simulink model "BDA_DynamicModel_pdg"  (R2021b)
settings: Solver=ode23t  StartTime=0.0  StopTime=10  FixedStep=0.000001  MaxStep=1e-5  MinStep=1e-7  RelTol=1e-3
undefined symbols (not defined in the file): X, Y, Z
libraries: sm_lib x47, nesl_utility x7, simulink x1
(part 2 of 3)

== matlab function BDA_DynamicModel_pdg/Modelo dinámico/h ==
  data: dq1 input; h output; dq2 input; dq3 input; dq4 input; dq5 input; dq6 input; q1 input; q2 input; q3 input; q4 input; q5 input; q6 input
function h = h(dq1,dq2,dq3,dq4,dq5,dq6,q1,q2,q3,q4,q5,q6)
%#codegen

%    This function was generated by the Symbolic Math Toolbox version 9.0.
%    01-Nov-2021 22:23:11

t2 = conj(dq1);
t3 = conj(dq2);
t4 = conj(dq3);
t5 = conj(dq4);
t6 = conj(dq5);
t7 = conj(dq6);
t8 = conj(q1);
t9 = conj(q2);
t10 = conj(q3);
t11 = conj(q4);
t12 = conj(q5);
t13 = conj(q6);
t14 = cos(q2);
t15 = cos(q4);
t16 = cos(q5);
t17 = cos(q6);
t18 = sin(q2);
t19 = sin(q4);
t20 = sin(q5);
t21 = sin(q6);
t22 = dq1+dq2;
t34 = dq5.*(3.0./5.0e+2);
t44 = dq3.*5.110348748545983e-1;
t51 = dq3.*8.595599785252598e-1;
t52 = dq5.*1.247162e-2;
t55 = 9.007199254740992e+15;
t56 = dq6.*9.99471e-3;
t58 = dq6.*1.838876e-2;
t60 = dq5.*5.68686e-3;
t63 = dq4.*5.84482e-3;
t67 = dq4.*6.47e-6;
t102 = dq3.*2.688673858077708e-3;
t103 = dq3.*2.986906857247653e-3;
t111 = dq3.*3.306395640309251e-6;
t23 = cos(t8);
t24 = cos(t9);
t25 = cos(t11);
t26 = cos(t12);
t27 = cos(t13);
t28 = sin(t8);
t29 = sin(t9);
t30 = sin(t11);
t31 = sin(t12);
t32 = sin(t13);
t33 = t2+t3;
t42 = t14.*1.051339e-1;
t43 = t18.*1.051339e-1;
t45 = t4.*5.110348748545983e-1;
t46 = t16.*5.110348748545983e-1;
t48 = t20.*5.110348748545983e-1;
t53 = t18.*3.235525e-2;
t54 = t4.*8.595599785252598e-1;
t59 = t14.*3.235525e-2;
t64 = t16.*t19.*8.595599785252598e-1;
t65 = t19.*t20.*8.595599785252598e-1;
t68 = t6.*4.36041e-5;
t69 = t6.*5.58e-9;
t70 = t6.*6.12e-9;
t71 = t6.*1.247162e-10;
t72 = t6.*5.68686e-11;
t73 = t6.*5.4e-10;
t75 = (q3.*t55)./9.007199254740992e+15;
t76 = (t10.*t55)./9.007199254740992e+15;
t81 = q3.*t55.*1.110223024625157e-16i;
t82 = t10.*t55.*1.110223024625157e-16i;
t104 = t7.*1.33637554986e-4;
t105 = t5.*1.688944904408e-4;
t106 = t7.*7.26350557185e-5;
t107 = t6.*6.1855407534e-5;
t109 = t6.*1.35652563578e-4;
t110 = t15.*t16.*4.990257941055339e-2;
t114 = t6.*7.732404399999999e-9;
t116 = t6.*3.5258532e-9;
t117 = t5.*1.869599668e-7;
t118 = t7.*1.87565352e-8;
t119 = t5.*4.57649406e-8;
t121 = t7.*1.01946042e-8;
t123 = t5.*6.36648e-11;
t124 = t5.*1.89372168e-8;
t125 = t5.*1.81773902e-8;
t127 = t6.*3.740375e-9;
t128 = t6.*3.2206632e-9;
t129 = t7.*1.96560591e-8;
t130 = t7.*1.09500687e-8;
t131 = t5.*2.01217e-11;
t132 = t5.*2.09628e-11;
t147 = t4.*8.974336263707516e-6;
t159 = t4.*8.631097478604537e-5;
t160 = t4.*3.253493310064303e-11;
t163 = t4.*2.338748069224912e-8;
t164 = t4.*9.289280326040201e-9;
t165 = t4.*2.957541243885479e-10;
t166 = t4.*9.554306323645785e-8;
t168 = t4.*1.344336929038854e-10;
t170 = t4.*4.301878172924333e-10;
t171 = t4.*9.677578217482396e-9;
t173 = t4.*1.028289044136177e-11;
t176 = t4.*1.071272187460197e-11;
t35 = t23.*t24.*(9.81e+2./1.0e+2);
t36 = t23.*t29.*(9.81e+2./1.0e+2);
t37 = t24.*t28.*(9.81e+2./1.0e+2);
t38 = t28.*t29.*(9.81e+2./1.0e+2);
t47 = -t43;
t49 = t24.*1.051339e-1;
t50 = t29.*1.051339e-1;
t61 = t24.*3.235525e-2;
t62 = t29.*3.235525e-2;
t66 = -t65;
t74 = -t71;
t77 = cos(t75);
t78 = sin(t75);
t79 = cos(t76);
t80 = sin(t76);
t83 = exp(t81);
t84 = -t81;
t85 = -t82;
t89 = exp(t82);
t112 = t42+t53;
t122 = t48+t64;
t39 = -t38;
t40 = t36+t37;
t57 = -t50;
t86 = 1.0./t83;
t87 = t15.*t77;
t88 = t19.*t77;
t90 = exp(t85);
t91 = t83-1.0;
t94 = t22.*t25.*t79;
t96 = t22.*t30.*t79;
t113 = t47+t59;
t115 = t49+t62;
t126 = t46+t66;
t133 = t77.*1.025512e-2;
t134 = t77.*1.273194e-2;
t135 = t77.*9.224950000000001e-3;
t143 = t22.*t79.*1.273194e-2;
t144 = t22.*t79.*1.025512e-2;
t145 = t22.*t79.*9.224950000000001e-3;
t180 = t83.*3.694216783411725e-1;
t181 = t83.*1.305783216588275e-1;
t183 = t89.*1.305783216588275e-1;
t184 = t89.*3.694216783411725e-1;
t188 = t33.*t77.*3.42298471896e-5;
t189 = t33.*t77.*3.07913148585e-5;
t190 = t33.*t77.*1.252822896e-7;
t191 = t33.*t77.*3.679077402936e-4;
t196 = t33.*t77.*2.2561264e-9;
t200 = t33.*t77.*1.5275005e-9;
t202 = t33.*t77.*2.029489e-9;
t203 = t33.*t77.*9.96910902e-8;
t204 = t33.*t77.*4.12514856e-8;
t208 = t33.*t77.*2.1020667e-9;
t226 = t15.*t55.*t78.*5.673626844500105e-17;
t227 = t19.*t55.*t78.*5.673626844500105e-17;
t228 = t16.*t55.*t78.*9.543032792050485e-17;
t229 = t20.*t55.*t78.*9.543032792050485e-17;
t232 = t22.*t55.*t80.*5.673626844500105e-17;
t233 = t22.*t55.*t80.*9.543032792050485e-17;
t234 = t15.*t55.*t78.*3.404176106700063e-19;
t236 = t33.*t55.*t78.*5.673626844500105e-17;
t237 = t33.*t55.*t78.*9.543032792050485e-17;
t239 = t83.*3.215186923359161e-3;
t241 = t83.*1.345257168956303e-2;
t242 = t89.*3.215186923359161e-3;
t243 = t89.*1.345257168956303e-2;
t247 = t55.*t78.*4.87211480085e-18;
t250 = t20.*t55.*t78.*9.537984527703491e-19;
t252 = t55.*t78.*5.577730892363251e-19;
t253 = t22.*t55.*t80.*4.87211480085e-18;
t254 = t20.*t55.*t78.*1.754845396851463e-18;
t255 = t15.*t55.*t78.*7.075931802640439e-19;
t256 = t15.*t55.*t78.*2.479366200131245e-18;
t258 = t15.*t55.*t78.*3.226512155691387e-19;
t259 = t20.*t55.*t78.*5.426989146380022e-19;
t260 = t19.*t55.*t78.*3.31613276532711e-19;
t261 = t16.*t55.*t78.*1.190170786299927e-18;
t262 = t15.*t55.*t78.*7.351481000981246e-18;
t263 = t19.*t55.*t78.*9.810473427588925e-18;
t264 = t19.*t55.*t78.*4.938358626738924e-18;
t265 = t22.*t55.*t80.*6.374153504905841e-18;
t270 = t16.*t55.*t78.*6.183885249248715e-21;
t272 = t20.*t55.*t78.*6.183885249248715e-21;
t273 = t55.*t78.*6.174342216456664e-22;
t274 = t22.*t55.*t80.*5.577730892363251e-19;
t275 = t15.*t55.*t78.*3.670836568391568e-22;
t278 = t22.*t55.*t80.*6.174342216456664e-22;
t304 = t33.*t55.*t78.*2.127584079327986e-20;
t309 = t33.*t55.*t78.*1.611765660673211e-20;
t310 = t55.*t78.*t112.*5.673626844500105e-17;
t312 = t33.*t55.*t78.*1.807184809125693e-24;
t313 = t33.*t55.*t78.*4.367363288720426e-24;
t314 = t33.*t55.*t78.*7.011568855396425e-25;
t316 = t33.*t55.*t78.*3.18707675245292e-25;
t317 = t33.*t55.*t78.*6.075552740993358e-27;
t318 = t33.*t55.*t78.*1.78416509397307e-23;
t319 = t33.*t55.*t78.*1.019864560784935e-24;
t322 = t33.*t55.*t78.*1.734674307524971e-24;
t326 = t33.*t55.*t78.*2.000486878131959e-27;
t331 = t33.*t55.*t78.*1.920220429318022e-27;
t393 = t2.*t55.*t78.*t112.*1.893760189037778e-19;
t400 = t2.*t55.*t78.*t112.*6.240989528950116e-24;
t402 = t2.*t55.*t78.*t112.*2.836813422250052e-24;
t408 = t2.*t55.*t78.*t112.*9.077802951200168e-24;
t41 = t35+t39;
t92 = t91.^2;
t93 = t90-1.0;
t95 = t33.*t87;
t97 = t33.*t88;
t98 = t88.*(3.0./5.0e+2);
t100 = -t96;
t108 = t96.*(3.0./5.0e+2);
t120 = t57+t61;
t136 = t88.*2.228474e-2;
t137 = t87.*4.539638e-2;
t138 = t88.*4.539638e-2;
t139 = t88.*1.247162e-2;
t140 = t88.*5.68686e-3;
t141 = t87.*5.84482e-3;
t142 = t87.*6.562549e-2;
t146 = t33.*t134;
t148 = t88.*6.47e-6;
t149 = t96.*2.228474e-2;
t151 = t94.*4.539638e-2;
t152 = t96.*4.539638e-2;
t154 = t96.*1.247162e-2;
t155 = t94.*5.84482e-3;
t156 = t94.*6.562549e-2;
t158 = t96.*5.68686e-3;
t161 = t96.*6.47e-6;
t182 = t86.*3.694216783411725e-1;
t185 = t86.*1.305783216588275e-1;
t186 = t90.*1.305783216588275e-1;
t187 = t90.*3.694216783411725e-1;
t230 = -t227;
t231 = -t228;
t235 = -t232;
t238 = -t236;
t240 = t86.*3.215186923359161e-3;
t244 = t86.*1.345257168956303e-2;
t245 = t90.*3.215186923359161e-3;
t246 = t90.*1.345257168956303e-2;
t248 = t40.*t55.*t80.*5.673626844500105e-17;
t257 = t33.*t247;
t266 = -t260;
t267 = -t261;
t268 = -t263;
t269 = -t264;
t271 = -t265;
t276 = -t275;
t277 = t44+t233;
t281 = t45+t237;
t297 = t40.*t55.*t80.*1.893760189037778e-19;
t299 = t88+t226;
t307 = -t304;
t311 = t55.*t78.*t113.*9.543032792050485e-17;
t320 = t2.*t310;
t321 = -t314;
t323 = -t316;
t324 = -t319;
t327 = dq1.*t55.*t80.*t115.*5.673626844500105e-17;
t328 = t2.*t55.*t78.*t113.*(-9.543032792050485e-17);
t397 = -t393;
t399 = t2.*t55.*t78.*t113.*3.185302114428987e-19;
t403 = -t400;
t404 = t2.*t55.*t78.*t113.*1.049733607125553e-23;
t407 = -t402;
t409 = t2.*t55.*t78.*t113.*4.771516396025242e-24;
t412 = t2.*t55.*t78.*t113.*1.526885246728078e-23;
t418 = -t408;
t99 = t93.^2;
t101 = -t97;
t150 = t97.*2.228474e-2;
t153 = -t148;
t157 = t95.*6.562549e-2;
t162 = t97.*4.36041e-5;
t167 = -t161;
t169 = t97.*5.58e-9;
t172 = t97.*6.12e-9;
t174 = t97.*1.247162e-10;
t175 = t97.*5.68686e-11;
t177 = t95.*6.562549e-10;
t178 = t97.*5.4e-10;
t192 = t95.*4.467003792e-7;
t193 = t95.*1.3117937708872e-3;
t194 = t97.*1.3117937708872e-3;
t195 = t97.*1.35652563578e-4;
t197 = t95.*5.75130288e-8;
t198 = t95.*1.688944904408e-4;
t199 = t97.*6.1855407534e-5;
t201 = t95.*7.13801892181e-4;
t205 = t97.*3.554536554e-7;
t206 = t97.*7.732404399999999e-9;
t207 = t97.*1.869599668e-7;
t209 = t97.*1.411827418e-7;
t210 = t97.*1.470842712e-7;
t211 = t97.*3.5258532e-9;
t213 = t97.*6.36648e-11;
t214 = t95.*3.74065293e-8;
t216 = t95.*1.928492118e-7;
t217 = t95.*1.601199586e-7;
t218 = t95.*2.6250196e-9;
t219 = t95.*1.57501176e-8;
t220 = t97.*3.740375e-9;
t221 = t97.*3.2206632e-9;
t222 = t97.*5.06601e-11;
t223 = t97.*2.09628e-11;
t249 = t41.*t55.*t80.*9.543032792050485e-17;
t251 = -t248;
t279 = dq4+t277;
t280 = t51+t235;
t282 = t5+t281;
t283 = t54+t238;
t298 = -t297;
t300 = t41.*t55.*t80.*3.185302114428987e-19;
t301 = t87+t230;
t302 = t17.*t299;
t303 = t21.*t299;
t315 = -t311;
t325 = t2.*t311;
t329 = -t327;
t330 = dq1.*t55.*t80.*t120.*9.543032792050485e-17;
t332 = t86.*t92.*7.997968101822611e-3;
t334 = t25.*t277.*1.273194e-2;
t335 = t30.*t277.*1.273194e-2;
t337 = t15.*t281.*1.273194e-2;
t338 = t19.*t281.*1.273194e-2;
t340 = t86.*t92.*5.407940120688672e-3;
t369 = t19.*t281.*1.273194e-10;
t388 = t16.*t299.*4.334075e-2;
t389 = t20.*t299.*4.334075e-2;
t406 = t19.*t281.*1.252822896e-7;
t414 = t15.*t281.*3.679077402936e-4;
t415 = t19.*t281.*3.679077402936e-4;
t417 = t19.*t281.*1.38484038186e-4;
t436 = t15.*t281.*9.96910902e-8;
t438 = t15.*t281.*3.95963334e-8;
t439 = t19.*t281.*3.95963334e-8;
t442 = t19.*t281.*7.257205800000001e-9;
t453 = t15.*t281.*4.12514856e-8;
t455 = t19.*t281.*4.12514856e-8;
t463 = t19.*t281.*5.092776e-10;
t465 = t19.*t281.*3.0556656e-9;
t484 = t86.*t92.*t112.*2.196325630278387e-1;
t495 = t86.*t92.*t113.*2.196325630278387e-1;
t509 = t2.*t86.*t92.*t113.*(-2.196325630278387e-1);
t521 = t2.*t86.*t92.*t112.*7.330961578512107e-4;
t528 = t2.*t86.*t92.*t113.*7.330961578512107e-4;
t529 = t2.*t86.*t92.*t112.*6.346599179580158e-3;
t537 = t2.*t86.*t92.*t112.*2.161184420193933e-6;
t538 = t2.*t86.*t92.*t112.*7.116095042101973e-7;
t539 = t2.*t86.*t92.*t112.*1.719722968507977e-6;
t540 = t2.*t86.*t92.*t112.*4.831916386612451e-8;
t541 = t2.*t86.*t92.*t112.*1.098162815139193e-8;
t542 = t2.*t86.*t92.*t113.*2.415958193306225e-8;
t543 = t2.*t86.*t92.*t113.*4.831916386612451e-8;
t544 = t2.*t86.*t92.*t112.*3.514121008445419e-8;
t547 = t2.*t86.*t92.*t113.*1.098162815139193e-8;
t555 = t180+t182+2.61156643317655e-1;
t556 = t181+t185+7.38843356682345e-1;
t557 = t183+t186+7.38843356682345e-1;
t558 = t184+t187+2.61156643317655e-1;
t714 = t257+t320+t328;
t777 = t147+t307+t397+t399;
t778 = t165+t321+t403+t404;
t779 = t168+t323+t407+t409;
t780 = t170+t324+t412+t418;
t179 = -t174;
t212 = -t207;
t215 = -t213;
t224 = -t222;
t225 = -t223;
t284 = t26.*t279;
t285 = t31.*t279;
t286 = t25.*t280;
t287 = t30.*t280;
t288 = t20.*t282;
t289 = t15.*t283;
t290 = t19.*t283;
t291 = t16.*t282;
t305 = t16.*t301;
t306 = t20.*t301;
t308 = -t303;
t333 = -t330;
t342 = -t335;
t343 = -t338;
t345 = t89.*t99.*7.997968101822611e-3;
t349 = t40.*t89.*t99.*2.196325630278387e-1;
t356 = t89.*t99.*5.407940120688672e-3;
t358 = t41.*t89.*t99.*2.196325630278387e-1;
t371 = -t369;
t386 = t303.*9.99471e-3;
t387 = t302.*1.838876e-2;
t401 = t40.*t89.*t99.*7.330961578512107e-4;
t405 = t41.*t89.*t99.*7.330961578512107e-4;
t411 = -t406;
t416 = t40.*t89.*t99.*6.346599179580158e-3;
t422 = -t415;
t423 = -t417;
t451 = -t439;
t456 = -t442;
t466 = -t455;
t477 = -t463;
t480 = -t465;
t501 = t2.*t484;
t503 = -t495;
t508 = t2.*t495;
t510 = dq1.*t89.*t99.*t115.*2.196325630278387e-1;
t511 = dq1.*t89.*t99.*t120.*2.196325630278387e-1;
t536 = -t528;
t548 = -t543;
t549 = -t542;
t553 = -t547;
t617 = t40.*t557;
t618 = t41.*t558;
t619 = t249+t251;
t620 = -t25.*(t248-t249);
t621 = -t30.*(t248-t249);
t633 = t112.*t556;
t634 = t113.*t555;
t635 = t25.*(t248-t249).*(-2.889644e-2);
t636 = t30.*(t248-t249).*(-2.889644e-2);
t640 = t30.*(t248-t249).*(-1.08769e-2);
t641 = dq1.*t115.*t557;
t643 = dq1.*t120.*t558;
t707 = t247+t310+t315;
t720 = t15.*t714;
t721 = t19.*t714;
t728 = t239+t240+t332+1.819229615328168e-2;
t729 = t241+t244+t340+9.510076620873934e-3;
t770 = t102+t271+t329+t330;
t796 = t277.*t778;
t797 = t277.*t779;
t798 = t280.*t779;
t799 = t280.*t780;
t292 = -t286;
t293 = -t289;
t294 = -t291;
t295 = t286.*(3.0./5.0e+2);
t336 = t285.*1.838876e-2;
t339 = t284.*1.247162e-2;
t341 = t285.*9.99471e-3;
t344 = t286.*2.228474e-2;
t347 = t286.*4.539638e-2;
t348 = t287.*4.539638e-2;
t350 = t285.*5.68686e-3;
t351 = t286.*1.247162e-2;
t352 = t284.*6.48e-5;
t353 = t286.*5.68686e-3;
t354 = t285.*6.48e-5;
t359 = -t349;
t360 = t289.*2.228474e-2;
t361 = t287.*5.84482e-3;
t362 = t287.*6.562549e-2;
t365 = t290.*6.562549e-2;
t366 = -t358;
t368 = t286.*6.47e-6;
t370 = t289.*4.36041e-5;
t373 = t289.*5.58e-9;
t375 = t289.*6.12e-9;
t376 = t289.*1.247162e-10;
t377 = t288.*5.68686e-11;
t378 = t289.*5.68686e-11;
t380 = t290.*6.562549e-10;
t381 = t289.*5.4e-10;
t385 = t288.*6.48e-13;
t390 = t305.*9.99471e-3;
t391 = t305.*1.838876e-2;
t392 = t306.*1.247162e-2;
t394 = t305.*5.68686e-3;
t395 = t305.*6.48e-5;
t396 = t306.*6.48e-5;
t410 = -t405;
t413 = t94+t287;
t419 = t290.*4.467003792e-7;
t420 = t289.*1.3117937708872e-3;
t421 = t290.*1.3117937708872e-3;
t424 = t95+t290;
t425 = t290.*5.75130288e-8;
t426 = t288.*7.26350557185e-5;
t427 = t290.*1.688944904408e-4;
t428 = t288.*6.1855407534e-5;
t430 = t289.*6.1855407534e-5;
t431 = t100+t286;
t432 = t291.*1.35652563578e-4;
t433 = t289.*1.35652563578e-4;
t434 = t288.*1.33637554986e-4;
t437 = t290.*7.13801892181e-4;
t443 = t101+t289;
t449 = t289.*3.554536554e-7;
t450 = t289.*7.732404399999999e-9;
t452 = t291.*7.0482312e-7;
t454 = t288.*7.0482312e-7;
t457 = t289.*1.470842712e-7;
t459 = t289.*3.5258532e-9;
t460 = t291.*7.1088234e-9;
t462 = t288.*3.2415102e-9;
t464 = t289.*1.869599668e-7;
t468 = t289.*1.411827418e-7;
t469 = t288.*4.0176e-11;
t470 = t288.*1.87565352e-8;
h = ft_1({dq1,dq5,dq6,t103,t104,t105,t106,t107,t108,t109,t110,t111,t112,t114,t116,t117,t118,t119,t121,t122,t123,t124,t125,t126,t127,t128,t129,t130,t131,t132,t133,t134,t135,t136,t137,t138,t139,t140,t141,t142,t143,t144,t145,t146,t149,t15,t150,t151,t152,t153,t154,t155,t156,t157,t158,t159,t16,t160,t162,t163,t164,t166,t167,t169,t17,t171,t172,t173,t174,t175,t176,t177,t178,t179,t188,t189,t19,t190,t191,t192,t193,t194,t195,t196,t197,t198,t199,t2,t20,t200,t201,t202,t203,t204,t205,t206,t208,t209,t21,t210,t211,t212,t214,t215,t216,t217,t218,t219,t22,t220,t221,t224,t225,t228,t229,t23,t231,t234,t24,t242,t243,t245,t246,t248,t249,t25,t250,t252,t253,t254,t255,t256,t258,t259,t26,t262,t266,t267,t268,t269,t27,t270,t272,t273,t274,t276,t277,t278,t279,t28,t280,t284,t285,t288,t289,t29,t290,t291,t292,t293,t294,t295,t297,t298,t299,t30,t300,t301,t302,t303,t305,t306,t308,t309,t31,t310,t312,t313,t315,t317,t318,t32,t322,t326,t327,t33,t331,t333,t334,t336,t337,t339,t34,t341,t342,t343,t344,t345,t347,t348,t349,t350,t351,t352,t353,t354,t356,t358,t359,t360,t361,t362,t365,t366,t368,t370,t371,t373,t375,t376,t377,t378,t380,t381,t385,t386,t387,t388,t389,t390,t391,t392,t394,t395,t396,t40,t401,t405,t41,t410,t411,t413,t414,t416,t419,t420,t421,t422,t423,t424,t425,t426,t427,t428,t43,t430,t432,t433,t434,t436,t437,t438,t449,t450,t451,t452,t453,t454,t456,t457,t459,t460,t462,t464,t466,t468,t469,t470,t477,t480,t484,t501,t503,t509,t510,t511,t52,t521,t529,t536,t537,t538,t539,t540,t541,t544,t548,t549,t55,t553,t56,t58,t59,t6,t60,t617,t618,t620,t621,t63,t633,t634,t635,t636,t640,t641,t643,t67,t68,t69,t70,t707,t71,t72,t720,t721,t728,t729,t73,t74,t77,t770,t777,t78,t79,t796,t797,t798,t799,t80,t96,t97,t98});
end
function h = ft_1(ct)
dq1 = ct{1};
dq5 = ct{2};
dq6 = ct{3};
t103 = ct{4};
t104 = ct{5};
t105 = ct{6};
t106 = ct{7};
t107 = ct{8};
t108 = ct{9};
t109 = ct{10};
t110 = ct{11};
t111 = ct{12};
t112 = ct{13};
t114 = ct{14};
t116 = ct{15};
t117 = ct{16};
t118 = ct{17};
t119 = ct{18};
t121 = ct{19};
t122 = ct{20};
t123 = ct{21};
t124 = ct{22};
t125 = ct{23};
t126 = ct{24};
t127 = ct{25};
t128 = ct{26};
t129 = ct{27};
t130 = ct{28};
t131 = ct{29};
t132 = ct{30};
t133 = ct{31};
t134 = ct{32};
t135 = ct{33};
t136 = ct{34};
t137 = ct{35};
t138 = ct{36};
t139 = ct{37};
t140 = ct{38};
t141 = ct{39};
t142 = ct{40};
t143 = ct{41};
t144 = ct{42};
t145 = ct{43};
t146 = ct{44};
t149 = ct{45};
t15 = ct{46};
t150 = ct{47};
t151 = ct{48};
t152 = ct{49};
t153 = ct{50};
t154 = ct{51};
t155 = ct{52};
t156 = ct{53};
t157 = ct{54};
t158 = ct{55};
t159 = ct{56};
t16 = ct{57};
t160 = ct{58};
t162 = ct{59};
t163 = ct{60};
t164 = ct{61};
t166 = ct{62};
t167 = ct{63};
t169 = ct{64};
t17 = ct{65};
t171 = ct{66};
t172 = ct{67};
t173 = ct{68};
t174 = ct{69};
t175 = ct{70};
t176 = ct{71};
t177 = ct{72};
t178 = ct{73};
t179 = ct{74};
t188 = ct{75};
t189 = ct{76};
t19 = ct{77};
t190 = ct{78};
t191 = ct{79};
t192 = ct{80};
t193 = ct{81};
t194 = ct{82};
t195 = ct{83};
t196 = ct{84};
t197 = ct{85};
t198 = ct{86};
t199 = ct{87};
t2 = ct{88};
t20 = ct{89};
t200 = ct{90};
t201 = ct{91};
t202 = ct{92};
t203 = ct{93};
t204 = ct{94};
t205 = ct{95};
t206 = ct{96};
t208 = ct{97};
t209 = ct{98};
t21 = ct{99};
t210 = ct{100};
t211 = ct{101};
t212 = ct{102};
t214 = ct{103};
t215 = ct{104};
t216 = ct{105};
t217 = ct{106};
t218 = ct{107};
t219 = ct{108};
t22 = ct{109};
t220 = ct{110};
t221 = ct{111};
t224 = ct{112};
t225 = ct{113};
t228 = ct{114};
t229 = ct{115};
t23 = ct{116};
t231 = ct{117};
t234 = ct{118};
t24 = ct{119};
t242 = ct{120};
t243 = ct{121};
t245 = ct{122};
t246 = ct{123};
t248 = ct{124};
t249 = ct{125};
t25 = ct{126};
t250 = ct{127};
t252 = ct{128};
t253 = ct{129};
t254 = ct{130};
t255 = ct{131};
t256 = ct{132};
t258 = ct{133};
t259 = ct{134};
t26 = ct{135};
t262 = ct{136};
t266 = ct{137};
t267 = ct{138};
t268 = ct{139};
t269 = ct{140};
t27 = ct{141};
t270 = ct{142};
t272 = ct{143};
t273 = ct{144};
t274 = ct{145};
t276 = ct{146};
t277 = ct{147};
t278 = ct{148};
t279 = ct{149};
t28 = ct{150};
t280 = ct{151};
t284 = ct{152};
t285 = ct{153};
t288 = ct{154};
t289 = ct{155};
t29 = ct{156};
t290 = ct{157};
t291 = ct{158};
t292 = ct{159};
t293 = ct{160};
t294 = ct{161};
t295 = ct{162};
t297 = ct{163};
t298 = ct{164};
t299 = ct{165};
t30 = ct{166};
t300 = ct{167};
t301 = ct{168};
t302 = ct{169};
t303 = ct{170};
t305 = ct{171};
t306 = ct{172};
t308 = ct{173};
t309 = ct{174};
t31 = ct{175};
t310 = ct{176};
t312 = ct{177};
t313 = ct{178};
t315 = ct{179};
t317 = ct{180};
t318 = ct{181};
t32 = ct{182};
t322 = ct{183};
t326 = ct{184};
t327 = ct{185};
t33 = ct{186};
t331 = ct{187};
t333 = ct{188};
t334 = ct{189};
t336 = ct{190};
t337 = ct{191};
t339 = ct{192};
t34 = ct{193};
t341 = ct{194};
t342 = ct{195};
t343 = ct{196};
t344 = ct{197};
t345 = ct{198};
t347 = ct{199};
t348 = ct{200};
t349 = ct{201};
t350 = ct{202};
t351 = ct{203};
t352 = ct{204};
t353 = ct{205};
t354 = ct{206};
t356 = ct{207};
t358 = ct{208};
t359 = ct{209};
t360 = ct{210};
t361 = ct{211};
t362 = ct{212};
t365 = ct{213};
t366 = ct{214};
t368 = ct{215};
t370 = ct{216};
t371 = ct{217};
t373 = ct{218};
t375 = ct{219};
t376 = ct{220};
t377 = ct{221};
t378 = ct{222};
t380 = ct{223};
t381 = ct{224};
t385 = ct{225};
t386 = ct{226};
t387 = ct{227};
t388 = ct{228};
t389 = ct{229};
t390 = ct{230};
t391 = ct{231};
t392 = ct{232};
t394 = ct{233};
t395 = ct{234};
t396 = ct{235};
t40 = ct{236};
t401 = ct{237};
t405 = ct{238};
t41 = ct{239};
t410 = ct{240};
t411 = ct{241};
t413 = ct{242};
t414 = ct{243};
t416 = ct{244};
t419 = ct{245};
t420 = ct{246};
t421 = ct{247};
t422 = ct{248};
t423 = ct{249};
t424 = ct{250};
t425 = ct{251};
t426 = ct{252};
t427 = ct{253};
t428 = ct{254};
t43 = ct{255};
t430 = ct{256};
t432 = ct{257};
t433 = ct{258};
t434 = ct{259};
t436 = ct{260};
t437 = ct{261};
t438 = ct{262};
t449 = ct{263};
t450 = ct{264};
t451 = ct{265};
t452 = ct{266};
t453 = ct{267};
t454 = ct{268};
t456 = ct{269};
t457 = ct{270};
t459 = ct{271};
t460 = ct{272};
t462 = ct{273};
t464 = ct{274};
t466 = ct{275};
t468 = ct{276};
t469 = ct{277};
t470 = ct{278};
t477 = ct{279};
t480 = ct{280};
t484 = ct{281};
t501 = ct{282};
t503 = ct{283};
t509 = ct{284};
t510 = ct{285};
t511 = ct{286};
t52 = ct{287};
t521 = ct{288};
t529 = ct{289};
t536 = ct{290};
t537 = ct{291};
t538 = ct{292};
t539 = ct{293};
t540 = ct{294};
t541 = ct{295};
t544 = ct{296};
t548 = ct{297};
t549 = ct{298};
t55 = ct{299};
t553 = ct{300};
t56 = ct{301};
t58 = ct{302};
t59 = ct{303};
t6 = ct{304};
t60 = ct{305};
t617 = ct{306};
t618 = ct{307};
t620 = ct{308};
t621 = ct{309};
t63 = ct{310};
t633 = ct{311};
t634 = ct{312};
t635 = ct{313};
t636 = ct{314};
t640 = ct{315};
t641 = ct{316};
t643 = ct{317};
t67 = ct{318};
t68 = ct{319};
t69 = ct{320};
t70 = ct{321};
t707 = ct{322};
t71 = ct{323};
t72 = ct{324};
t720 = ct{325};
t721 = ct{326};
t728 = ct{327};
t729 = ct{328};
t73 = ct{329};
t74 = ct{330};
t77 = ct{331};
t770 = ct{332};
t777 = ct{333};
t78 = ct{334};
t79 = ct{335};
t796 = ct{336};
t797 = ct{337};
t798 = ct{338};
t799 = ct{339};
t80 = ct{340};
t96 = ct{341};
t97 = ct{342};
t98 = ct{343};
t471 = t290.*3.74065293e-8;
t474 = t288.*1.01946042e-8;
t478 = t289.*6.36648e-11;
t479 = t291.*3.6936e-11;
t482 = t291.*4.988648e-10;
t483 = t290.*2.6250196e-9;
t485 = t288.*1.3648464e-9;
t488 = t288.*2.274744e-10;
t489 = t290.*1.928492118e-7;
t490 = t290.*1.601199586e-7;
t491 = t291.*2.592e-12;
t493 = t288.*2.592e-12;
t494 = t289.*3.2206632e-9;
t496 = t288.*1.96560591e-8;
t497 = t288.*1.09500687e-8;
t498 = t288.*1.5552e-11;
t499 = t289.*3.740375e-9;
t500 = t290.*1.57501176e-8;
t504 = t289.*2.09628e-11;
t506 = t289.*5.06601e-11;
t512 = -t511;
t513 = t291.*2.9925408e-9;
t514 = t288.*2.268264e-10;
t515 = t291.*8.454019999999999e-11;
t622 = t229+t305;
t623 = t231+t306;
t624 = -t17.*(t228-t306);
t625 = -t21.*(t228-t306);
t628 = t617.*3.33783e-3;
t629 = t618.*3.33783e-3;
t630 = t618.*2.889644e-2;
t637 = t2.*t633;
t638 = -t634;
t639 = t2.*t634;
t644 = t17.*(t228-t306).*(-9.99471e-3);
t645 = t21.*(t228-t306).*(-1.838876e-2);
t646 = t17.*(t228-t306).*9.99471e-3;
t647 = -t643;
t703 = -t26.*(t349-t618);
t704 = -t25.*(t358-t617);
t705 = -t30.*(t358-t617);
t706 = t30.*(t358-t617);
t708 = t15.*t707;
t709 = t19.*t707;
t712 = t25.*(t358-t617).*(-2.889644e-2);
t715 = t25.*(t358-t617).*(-1.08769e-2);
t716 = t31.*(t349-t618).*(-7.26735e-3);
t717 = t26.*(t349-t618).*(-1.08769e-2);
t718 = t31.*(t349-t618).*(-1.08769e-2);
t719 = t253+t327+t333;
t722 = -t721;
t726 = t721./1.0e+8;
t730 = t15.*t728;
t731 = t19.*t728;
t732 = t242+t245+t345+1.819229615328168e-2;
t733 = t243+t246+t356+9.510076620873934e-3;
t734 = t33.*t728;
t735 = t33.*t729;
t738 = t720.*2.889644e-2;
t739 = t721.*2.889644e-2;
t740 = t721.*1.08769e-2;
t741 = t721.*9.840000000000001e-6;
t745 = t720.*3.24e-6;
t746 = t721.*5.7e-7;
t747 = t721.*3.24e-6;
t748 = t720.*7.83e-6;
t749 = t720.*3.11e-6;
t750 = t721.*3.11e-6;
t753 = t721.*2.4e-7;
t756 = t721.*4.0e-8;
t773 = t134+t729;
t788 = t27.*(t30.*(t248-t249)+t25.*(t358-t617)).*(-7.26735e-3);
t789 = t32.*(t30.*(t248-t249)+t25.*(t358-t617)).*(-7.26735e-3);
t790 = t32.*(t30.*(t248-t249)+t25.*(t358-t617)).*7.26735e-3;
t800 = t503+t633+t728;
t296 = -t295;
t346 = -t339;
t355 = -t344;
t357 = -t347;
t363 = -t351;
t364 = -t353;
t367 = -t360;
t372 = -t370;
t374 = -t373;
t379 = -t375;
t382 = -t376;
t383 = -t378;
t384 = -t381;
t398 = -t396;
t429 = -t420;
t435 = -t430;
t440 = -t432;
t441 = -t433;
t444 = dq5+t96+t292;
t445 = t26.*t413;
t446 = t16.*t424;
t447 = t31.*t413;
t448 = t20.*t424;
t458 = -t449;
t461 = -t450;
t467 = t6+t97+t293;
t473 = -t457;
t475 = -t459;
t476 = -t460;
t481 = -t468;
t492 = -t482;
t502 = -t494;
t507 = -t499;
t516 = -t513;
t517 = -t515;
t525 = t26.*(t96+t292).*(-4.334075e-2);
t526 = t31.*(t96+t292).*(-4.334075e-2);
t527 = t20.*(t97+t293).*(-4.334075e-2);
t532 = t26.*(t96+t292).*4.334075e-2;
t534 = t31.*(t96+t292).*4.334075e-2;
t535 = t20.*(t97+t293).*4.334075e-2;
t545 = t16.*(t97+t293).*(-4.334075e-10);
t546 = t20.*(t97+t293).*(-4.334075e-10);
t551 = t16.*(t97+t293).*4.334075e-10;
t552 = t20.*(t97+t293).*4.334075e-10;
t563 = t16.*(t97+t293).*(-4.71413003675e-4);
t564 = t20.*(t97+t293).*(-4.71413003675e-4);
t565 = t16.*(t97+t293).*4.71413003675e-4;
t566 = t20.*(t97+t293).*4.71413003675e-4;
t567 = t16.*(t97+t293).*(-3.149723995125e-4);
t570 = t16.*(t97+t293).*3.149723995125e-4;
t577 = t16.*(t97+t293).*(-2.47042275e-8);
t580 = t16.*(t97+t293).*(-2.6871265e-8);
t582 = t20.*(t97+t293).*(-2.6871265e-8);
t585 = t16.*(t97+t293).*(-4.4207565e-8);
t586 = t16.*(t97+t293).*(-4.03068975e-8);
t587 = t16.*(t97+t293).*2.47042275e-8;
t589 = t16.*(t97+t293).*2.6871265e-8;
t591 = t20.*(t97+t293).*2.6871265e-8;
t594 = t20.*(t97+t293).*(-1.040178e-8);
t595 = t16.*(t97+t293).*4.4207565e-8;
t596 = t16.*(t97+t293).*4.03068975e-8;
t600 = t16.*(t97+t293).*(-1.73363e-9);
t601 = t16.*(t97+t293).*(-3.9006675e-9);
t602 = t20.*(t97+t293).*(-1.73363e-9);
t604 = t20.*(t97+t293).*1.040178e-8;
t605 = t16.*(t97+t293).*1.73363e-9;
t606 = t16.*(t97+t293).*3.9006675e-9;
t607 = t20.*(t97+t293).*1.73363e-9;
t626 = t17.*t622.*(3.0./5.0e+2);
t627 = t21.*t622.*(3.0./5.0e+2);
t631 = -t629;
t632 = -t630;
t642 = t2.*t638;
t648 = t637.*3.33783e-3;
t649 = t639.*3.33783e-3;
t650 = t639.*2.889644e-2;
t652 = t639.*9.840000000000001e-6;
t655 = t637.*1.1e-7;
t656 = t637.*2.2e-7;
t657 = t639.*2.2e-7;
t659 = t639.*3.24e-6;
t660 = t637.*5.0e-8;
t661 = t639.*7.83e-6;
t662 = t639.*5.0e-8;
t663 = t639.*1.6e-7;
t699 = t302+t625;
t700 = t308+t624;
t701 = t366+t617;
t702 = t359+t618;
t710 = -t709;
t711 = t706.*(-2.889644e-2);
t713 = t706.*2.889644e-2;
t723 = t30.*t719;
t724 = t25.*t719;
t727 = -t726;
t736 = t22.*t732;
t737 = t22.*t733;
t742 = -t739;
t743 = -t740;
t744 = -t741;
t751 = -t746;
t752 = -t747;
t754 = -t750;
t755 = -t753;
t757 = -t756;
t758 = t734.*3.33783e-3;
t759 = t735.*3.33783e-3;
t760 = t735.*2.889644e-2;
t761 = t735.*9.840000000000001e-6;
t762 = t734.*1.1e-7;
t763 = t734.*2.2e-7;
t764 = t735.*2.2e-7;
t765 = t735.*3.24e-6;
t766 = t735.*7.83e-6;
t767 = t734.*5.0e-8;
t768 = t735.*5.0e-8;
t769 = t735.*1.6e-7;
t774 = t20.*t773;
t775 = t16.*t773;
t781 = t136+t262+t731;
t782 = t142+t268+t730;
t785 = t621+t704;
t786 = t620+t706;
t787 = -t31.*(t705+t25.*(t248-t249));
t791 = t26.*(t705+t25.*(t248-t249)).*(-7.26735e-3);
t792 = t26.*(t705+t25.*(t248-t249)).*(-1.08769e-2);
t793 = t31.*(t705+t25.*(t248-t249)).*(-1.08769e-2);
t794 = t26.*(t705+t25.*(t248-t249)).*7.26735e-3;
t795 = t26.*(t705+t25.*(t248-t249)).*1.08769e-2;
t801 = t15.*t800;
t802 = t19.*t800;
t803 = t509+t637+t734;
t822 = t484+t638+t773;
t863 = t27.*(t31.*(t705+t25.*(t248-t249))+t26.*(t349-t618)).*(-7.26735e-3);
t864 = t32.*(t31.*(t705+t25.*(t248-t249))+t26.*(t349-t618)).*(-7.26735e-3);
t472 = -t447;
t486 = t27.*t444;
t487 = t32.*t444;
t518 = t447.*1.247162e-2;
t519 = t445.*9.99471e-3;
t520 = t445.*1.838876e-2;
t522 = t445.*5.68686e-3;
t523 = t445.*6.48e-5;
t524 = t447.*6.48e-5;
t550 = t446.*5.68686e-11;
t554 = t446.*6.48e-13;
t559 = t448.*1.35652563578e-4;
t560 = t446.*1.33637554986e-4;
t561 = t446.*7.26350557185e-5;
t562 = t446.*6.1855407534e-5;
t568 = t446.*7.0482312e-7;
t569 = t448.*7.0482312e-7;
t571 = t448.*7.1088234e-9;
t572 = t446.*3.2415102e-9;
t574 = t446.*4.0176e-11;
t575 = t446.*1.87565352e-8;
t576 = t21.*t467.*7.26350557185e-5;
t578 = t446.*1.01946042e-8;
t579 = t17.*t467.*1.33637554986e-4;
t581 = t448.*3.6936e-11;
t583 = t448.*4.988648e-10;
t584 = t446.*1.3648464e-9;
t588 = t446.*2.274744e-10;
t592 = t446.*2.592e-12;
t593 = t448.*2.592e-12;
t597 = t446.*1.96560591e-8;
t598 = t446.*1.09500687e-8;
t599 = t446.*1.5552e-11;
t608 = t21.*t467.*1.01946042e-8;
t609 = t21.*t467.*9.2950803e-9;
t610 = t17.*t467.*1.71015468e-8;
t611 = t17.*t467.*1.87565352e-8;
t612 = t21.*t467.*8.995239e-10;
t613 = t17.*t467.*1.6549884e-9;
t614 = t446.*2.268264e-10;
t615 = t448.*2.9925408e-9;
t616 = t448.*8.454019999999999e-11;
t651 = -t649;
t653 = -t650;
t654 = -t652;
t658 = -t657;
t664 = -t659;
t665 = -t661;
t666 = -t662;
t667 = -t663;
t668 = t285+t445;
t670 = t288+t446;
t672 = t294+t448;
t687 = t21.*(t291-t448).*(-1.33637554986e-4);
t688 = t17.*(t291-t448).*(-7.26350557185e-5);
t689 = t17.*(t291-t448).*7.26350557185e-5;
t690 = t17.*(t291-t448).*(-1.01946042e-8);
t691 = t17.*(t291-t448).*(-9.2950803e-9);
t692 = t21.*(t291-t448).*(-1.71015468e-8);
t693 = t21.*(t291-t448).*(-1.87565352e-8);
t694 = t21.*(t291-t448).*(-1.6549884e-9);
t695 = t17.*(t291-t448).*1.01946042e-8;
t696 = t17.*(t291-t448).*9.2950803e-9;
t697 = t17.*(t291-t448).*(-8.995239e-10);
t698 = t17.*(t291-t448).*8.995239e-10;
t725 = -t723;
t776 = -t774;
t783 = t16.*t781;
t784 = t20.*t781;
t804 = t15.*t803;
t805 = t19.*t803;
t806 = t512+t641+t736;
t823 = t16.*t822;
t824 = t20.*t822;
t826 = t146+t501+t642+t735;
t829 = t144+t510+t647+t737;
t830 = t143+t510+t647+t737;
t858 = t189+t536+t648+t758;
t860 = t703+t787;
t861 = t202+t548+t656+t763;
t870 = t136+t256+t708+t802;
t873 = t142+t269+t710+t801;
t505 = -t486;
t530 = -t524;
t531 = t487.*9.99471e-3;
t533 = t486.*1.838876e-2;
t573 = -t569;
t590 = -t581;
t603 = -t593;
t669 = dq6+t668;
t671 = t284+t472;
t675 = t27.*t668.*(3.0./5.0e+2);
t676 = t32.*t668.*(3.0./5.0e+2);
t680 = t21.*t670.*4.36041e-5;
t681 = t17.*t670.*4.36041e-5;
t682 = t21.*t670.*5.58e-9;
t683 = t17.*t670.*6.12e-9;
t684 = t21.*t670.*6.12e-9;
t685 = t21.*t670.*5.4e-10;
t686 = t17.*t670.*5.4e-10;
t807 = t25.*t806;
t808 = t30.*t806;
t809 = t804./1.0e+8;
t810 = t804.*2.889644e-2;
t811 = t805.*2.889644e-2;
t812 = t804.*1.08769e-2;
t813 = t804.*9.840000000000001e-6;
t814 = t804.*5.7e-7;
t815 = t804.*3.24e-6;
t816 = t805.*3.24e-6;
t817 = t805.*7.83e-6;
t818 = t804.*3.11e-6;
t819 = t805.*3.11e-6;
t820 = t804.*2.4e-7;
t821 = t804.*4.0e-8;
t825 = -t824;
t827 = t16.*t826;
t828 = t145+t806;
t831 = t26.*t830;
t832 = t31.*t830;
t835 = (t20.*t826)./1.0e+8;
t839 = t20.*t826.*1.08769e-2;
t840 = t20.*t826.*7.26735e-3;
t843 = t20.*t826.*5.7e-7;
t844 = t20.*t826.*9.3e-7;
t845 = t20.*t826.*1.02e-6;
t847 = t20.*t826.*6.2e-7;
t853 = t20.*t826.*9.0e-8;
t855 = t20.*t826.*4.0e-8;
t859 = t188+t521+t651+t759;
t862 = t196+t540+t658+t764;
t865 = t22.*t79.*t861;
t868 = t389+t775+t784;
t869 = t155+t167+t361+t368+t830;
t871 = t16.*t870;
t872 = t20.*t870;
t876 = t777.*t829;
t877 = t770.*t858;
t880 = t191+t198+t212+t427+t464+t529+t653+t760;
t881 = t190+t197+t215+t425+t478+t537+t654+t761;
t882 = t150+t337+t367+t720+t805;
t884 = t157+t343+t365+t722+t804;
t917 = t829.*t858;
t919 = t200+t541+t549+t655+t666+t762+t768;
t920 = t208+t544+t553+t660+t667+t767+t769;
t673 = t27.*t671;
t674 = t32.*t671;
t833 = -t832;
t834 = t827./1.0e+8;
t837 = -t835;
t838 = t827.*1.08769e-2;
t841 = -t839;
t842 = -t840;
t846 = t827.*6.2e-7;
t848 = -t843;
t849 = -t844;
t850 = -t845;
t851 = t827.*2.4e-7;
t852 = -t847;
t854 = t827.*4.0e-8;
t856 = -t853;
t857 = -t855;
t866 = t22.*t79.*t862;
t874 = t777.*t828;
t875 = t770.*t859;
t878 = -t876;
t879 = -t877;
t883 = t20.*t882;
t885 = t149+t334+t355+t724+t808;
t886 = (t16.*t882)./1.0e+8;
t890 = t156+t342+t362+t725+t807;
t894 = t16.*t882.*1.08769e-2;
t896 = t16.*t882.*7.26735e-3;
t897 = t16.*t882.*5.7e-7;
t898 = t16.*t882.*9.3e-7;
t899 = t16.*t882.*1.02e-6;
t900 = t16.*t882.*6.2e-7;
t903 = t17.*t884.*7.26735e-3;
t904 = t21.*t884.*7.26735e-3;
t905 = t16.*t882.*9.0e-8;
t906 = t16.*t882.*4.0e-8;
t908 = t17.*t884.*1.02e-6;
t909 = t21.*t884.*9.3e-7;
t910 = t21.*t884.*1.02e-6;
t911 = t17.*t884.*9.0e-8;
t912 = t21.*t884.*9.0e-8;
t913 = t413.*t881;
t914 = t63+t103+t152+t274+t334+t357+t724+t808;
t915 = t67+t111+t151+t278+t342+t348+t725+t807;
t916 = t828.*t859;
t921 = t105+t159+t194+t309+t414+t429+t738+t811;
t922 = t117+t166+t193+t318+t421+t422+t742+t810;
t923 = t123+t160+t192+t317+t411+t419+t744+t813;
t924 = t119+t163+t205+t313+t436+t458+t748+t817;
t925 = t124+t171+t210+t312+t453+t473+t745+t816;
t926 = t125+t164+t209+t322+t438+t481+t749+t819;
t927 = t277.*t919;
t928 = t280.*t920;
t937 = t797+t799+t865;
t940 = t389+t823+t872;
t941 = t201+t423+t428+t437+t440+t559+t562+t743+t812;
t942 = t214+t456+t462+t471+t476+t571+t572+t751+t814;
t943 = t218+t477+t483+t488+t492+t583+t588+t757+t821;
t961 = t132+t176+t203+t216+t224+t326+t466+t489+t506+t539+t665+t752+t766+t815;
t962 = t131+t173+t204+t217+t225+t331+t451+t490+t504+t538+t664+t754+t765+t818;
t677 = t674.*1.838876e-2;
t678 = t673.*9.99471e-3;
t771 = t487+t673;
t772 = t505+t674;
t836 = -t834;
t867 = -t866;
t887 = t883./1.0e+8;
t888 = t31.*t885;
t891 = t26.*t885;
t892 = t27.*t890;
t893 = t32.*t890;
t895 = t883.*1.08769e-2;
t901 = t883.*6.2e-7;
t902 = t883.*2.4e-7;
t907 = t883.*4.0e-8;
t918 = -t916;
t929 = t279.*t925;
t930 = t279.*t926;
t931 = t413.*t923;
t933 = -t924.*(t96+t292);
t934 = -t925.*(t96+t292);
t935 = t346+t350+t518+t522+t890;
t939 = t55.*t78.*t937.*9.543032792050485e-17;
t944 = t535+t827+t883;
t959 = t671.*t942;
t960 = t671.*t943;
t964 = t401+t631+t874+t879;
t965 = t410+t628+t875+t878;
t967 = t869.*t921;
t968 = t880.*t914;
t970 = t869.*t922;
t971 = t880.*t915;
t974 = t279.*t962;
t975 = -t961.*(t96+t292);
t977 = t107+t199+t435+t452+t565+t573+t841+t894;
t982 = t914.*t922;
t983 = t915.*t921;
t987 = t927+t928;
t990 = t68+t162+t372+t570+t576+t579+t687+t689+t842+t896;
t991 = t69+t169+t374+t596+t609+t610+t692+t696+t849+t898;
t992 = t70+t172+t379+t595+t608+t611+t693+t695+t850+t899;
t993 = t73+t178+t384+t606+t612+t613+t694+t698+t856+t905;
t1007 = t116+t177+t211+t371+t377+t380+t475+t517+t550+t589+t616+t727+t809+t852+t900;
t1008 = t72+t175+t219+t383+t480+t485+t500+t516+t551+t584+t615+t755+t820+t837+t886;
t679 = -t677;
t889 = -t887;
t932 = -t931;
t936 = t796+t798+t867;
t945 = t534+t831+t888;
t949 = t17.*t944.*7.26735e-3;
t950 = t21.*t944.*7.26735e-3;
t952 = t17.*t944.*9.3e-7;
t953 = t17.*t944.*1.02e-6;
t954 = t21.*t944.*1.02e-6;
t956 = t17.*t944.*9.0e-8;
t957 = t21.*t944.*9.0e-8;
t966 = t60+t158+t352+t364+t530+t532+t833+t891;
t969 = -t968;
t972 = -t971;
t973 = t71+t174+t382+t385+t552+t554+t834+t887;
t976 = t109+t195+t441+t454+t566+t568+t838+t895;
t978 = t114+t206+t461+t469+t574+t591+t846+t901;
t984 = -t983;
t986 = t298+t300+t917+t918;
t988 = t77.*t987;
t994 = -t991.*(t486-t674);
t995 = t771.*t992;
t996 = t771.*t993;
t997 = -t993.*(t486-t674);
t1010 = t444.*t1007;
t1012 = t935.*t977;
t1017 = t668.*t1008;
t1019 = t913+t930+t934;
t1023 = t55.*t78.*(-t929+t931+t924.*(t96+t292)).*(-9.543032792050485e-17);
t1024 = t55.*t78.*(-t929+t931+t924.*(t96+t292)).*9.543032792050485e-17;
t1025 = t127+t220+t479+t493+t507+t587+t590+t592+t607+t848+t854+t897+t907;
t1026 = t128+t221+t491+t498+t502+t599+t603+t604+t605+t851+t857+t902+t906;
t1030 = t974+t975;
t938 = t55.*t78.*t936.*5.673626844500105e-17;
t946 = t27.*t945;
t947 = t32.*t945;
t951 = -t950;
t955 = -t954;
t958 = -t957;
h = ft_2({dq1,t1010,t1012,t1017,t1019,t1024,t1025,t1026,t1030,t104,t106,t108,t110,t112,t118,t121,t122,t126,t129,t130,t133,t135,t137,t138,t139,t140,t141,t15,t153,t154,t16,t17,t179,t19,t2,t20,t21,t218,t228,t23,t234,t24,t248,t249,t25,t250,t252,t254,t255,t258,t259,t26,t266,t267,t27,t270,t272,t273,t276,t28,t29,t292,t296,t297,t299,t30,t300,t301,t303,t306,t31,t310,t315,t32,t336,t34,t341,t349,t354,t358,t363,t376,t386,t387,t388,t390,t391,t392,t394,t395,t398,t40,t405,t41,t416,t426,t43,t434,t444,t470,t474,t477,t483,t484,t486,t492,t496,t497,t514,t519,t52,t520,t523,t531,t532,t533,t546,t55,t56,t560,t561,t575,t578,t58,t583,t59,t597,t598,t614,t617,t618,t622,t626,t627,t628,t632,t635,t636,t638,t640,t645,t646,t668,t669,t671,t674,t675,t676,t678,t679,t680,t681,t682,t683,t684,t685,t686,t699,t705,t706,t708,t710,t712,t713,t715,t716,t717,t718,t728,t729,t730,t731,t74,t757,t771,t773,t776,t78,t782,t783,t788,t790,t793,t794,t795,t796,t797,t798,t799,t80,t800,t801,t802,t821,t822,t825,t833,t836,t863,t864,t865,t866,t868,t871,t873,t875,t876,t889,t891,t892,t893,t903,t904,t908,t909,t910,t911,t912,t916,t917,t924,t929,t931,t932,t933,t935,t938,t939,t940,t941,t945,t946,t947,t949,t951,t952,t953,t955,t956,t958,t959,t96,t960,t964,t966,t967,t968,t969,t970,t971,t972,t973,t976,t977,t978,t98,t982,t984,t988,t990,t991,t994,t995,t996,t997});
end
function h = ft_2(ct)
dq1 = ct{1};
t1010 = ct{2};
t1012 = ct{3};
t1017 = ct{4};
t1019 = ct{5};
t1024 = ct{6};
t1025 = ct{7};
t1026 = ct{8};
t1030 = ct{9};
t104 = ct{10};
t106 = ct{11};
t108 = ct{12};
t110 = ct{13};
t112 = ct{14};
t118 = ct{15};
t121 = ct{16};
t122 = ct{17};
t126 = ct{18};
t129 = ct{19};
t130 = ct{20};
t133 = ct{21};
t135 = ct{22};
t137 = ct{23};
t138 = ct{24};
t139 = ct{25};
t140 = ct{26};
t141 = ct{27};
t15 = ct{28};
t153 = ct{29};
t154 = ct{30};
t16 = ct{31};
t17 = ct{32};
t179 = ct{33};
t19 = ct{34};
t2 = ct{35};
t20 = ct{36};
t21 = ct{37};
t218 = ct{38};
t228 = ct{39};
t23 = ct{40};
t234 = ct{41};
t24 = ct{42};
t248 = ct{43};
t249 = ct{44};
t25 = ct{45};
t250 = ct{46};
t252 = ct{47};
t254 = ct{48};
t255 = ct{49};
t258 = ct{50};
t259 = ct{51};
t26 = ct{52};
t266 = ct{53};
t267 = ct{54};
t27 = ct{55};
t270 = ct{56};
t272 = ct{57};
t273 = ct{58};
t276 = ct{59};
t28 = ct{60};
t29 = ct{61};
t292 = ct{62};
t296 = ct{63};
t297 = ct{64};
t299 = ct{65};
t30 = ct{66};
t300 = ct{67};
t301 = ct{68};
t303 = ct{69};
t306 = ct{70};
t31 = ct{71};
t310 = ct{72};
t315 = ct{73};
t32 = ct{74};
t336 = ct{75};
t34 = ct{76};
t341 = ct{77};
t349 = ct{78};
t354 = ct{79};
t358 = ct{80};
t363 = ct{81};
t376 = ct{82};
t386 = ct{83};
t387 = ct{84};
t388 = ct{85};
t390 = ct{86};
t391 = ct{87};
t392 = ct{88};
t394 = ct{89};
t395 = ct{90};
t398 = ct{91};
t40 = ct{92};
t405 = ct{93};
t41 = ct{94};
t416 = ct{95};
t426 = ct{96};
t43 = ct{97};
t434 = ct{98};
t444 = ct{99};
t470 = ct{100};
t474 = ct{101};
t477 = ct{102};
t483 = ct{103};
t484 = ct{104};
t486 = ct{105};
t492 = ct{106};
t496 = ct{107};
t497 = ct{108};
t514 = ct{109};
t519 = ct{110};
t52 = ct{111};
t520 = ct{112};
t523 = ct{113};
t531 = ct{114};
t532 = ct{115};
t533 = ct{116};
t546 = ct{117};
t55 = ct{118};
t56 = ct{119};
t560 = ct{120};
t561 = ct{121};
t575 = ct{122};
t578 = ct{123};
t58 = ct{124};
t583 = ct{125};
t59 = ct{126};
t597 = ct{127};
t598 = ct{128};
t614 = ct{129};
t617 = ct{130};
t618 = ct{131};
t622 = ct{132};
t626 = ct{133};
t627 = ct{134};
t628 = ct{135};
t632 = ct{136};
t635 = ct{137};
t636 = ct{138};
t638 = ct{139};
t640 = ct{140};
t645 = ct{141};
t646 = ct{142};
t668 = ct{143};
t669 = ct{144};
t671 = ct{145};
t674 = ct{146};
t675 = ct{147};
t676 = ct{148};
t678 = ct{149};
t679 = ct{150};
t680 = ct{151};
t681 = ct{152};
t682 = ct{153};
t683 = ct{154};
t684 = ct{155};
t685 = ct{156};
t686 = ct{157};
t699 = ct{158};
t705 = ct{159};
t706 = ct{160};
t708 = ct{161};
t710 = ct{162};
t712 = ct{163};
t713 = ct{164};
t715 = ct{165};
t716 = ct{166};
t717 = ct{167};
t718 = ct{168};
t728 = ct{169};
t729 = ct{170};
t730 = ct{171};
t731 = ct{172};
t74 = ct{173};
t757 = ct{174};
t771 = ct{175};
t773 = ct{176};
t776 = ct{177};
t78 = ct{178};
t782 = ct{179};
t783 = ct{180};
t788 = ct{181};
t790 = ct{182};
t793 = ct{183};
t794 = ct{184};
t795 = ct{185};
t796 = ct{186};
t797 = ct{187};
t798 = ct{188};
t799 = ct{189};
t80 = ct{190};
t800 = ct{191};
t801 = ct{192};
t802 = ct{193};
t821 = ct{194};
t822 = ct{195};
t825 = ct{196};
t833 = ct{197};
t836 = ct{198};
t863 = ct{199};
t864 = ct{200};
t865 = ct{201};
t866 = ct{202};
t868 = ct{203};
t871 = ct{204};
t873 = ct{205};
t875 = ct{206};
t876 = ct{207};
t889 = ct{208};
t891 = ct{209};
t892 = ct{210};
t893 = ct{211};
t903 = ct{212};
t904 = ct{213};
t908 = ct{214};
t909 = ct{215};
t910 = ct{216};
t911 = ct{217};
t912 = ct{218};
t916 = ct{219};
t917 = ct{220};
t924 = ct{221};
t929 = ct{222};
t931 = ct{223};
t932 = ct{224};
t933 = ct{225};
t935 = ct{226};
t938 = ct{227};
t939 = ct{228};
t940 = ct{229};
t941 = ct{230};
t945 = ct{231};
t946 = ct{232};
t947 = ct{233};
t949 = ct{234};
t951 = ct{235};
t952 = ct{236};
t953 = ct{237};
t955 = ct{238};
t956 = ct{239};
t958 = ct{240};
t959 = ct{241};
t96 = ct{242};
t960 = ct{243};
t964 = ct{244};
t966 = ct{245};
t967 = ct{246};
t968 = ct{247};
t969 = ct{248};
t970 = ct{249};
t971 = ct{250};
t972 = ct{251};
t973 = ct{252};
t976 = ct{253};
t977 = ct{254};
t978 = ct{255};
t98 = ct{256};
t982 = ct{257};
t984 = ct{258};
t988 = ct{259};
t990 = ct{260};
t991 = ct{261};
t994 = ct{262};
t995 = ct{263};
t996 = ct{264};
t997 = ct{265};
t963 = t52+t154+t354+t363+t523+t945;
t979 = t444.*t973;
t980 = t444.*t978;
t985 = t34+t108+t296+t531+t532+t533+t678+t679+t833+t891;
t989 = -t988;
t1000 = t106+t426+t561+t680+t904+t949;
t1002 = t121+t474+t578+t684+t910+t953;
t1009 = t74+t179+t218+t376+t477+t483+t492+t514+t546+t583+t614+t757+t821+t836+t889;
t1011 = t935.*t976;
t1015 = t941.*t966;
t1020 = t299.*t1019;
t1022 = t929+t932+t933;
t1028 = t966.*t976;
t1031 = t301.*t1030;
t1033 = t671.*t1025;
t1034 = t668.*t1026;
t1035 = t636+t712+t967+t969;
t1036 = t635+t713+t970+t972;
t1037 = t416+t632+t982+t984;
t1057 = t960+t1010+t1017;
t948 = -t947;
t981 = -t980;
t998 = t56+t341+t519+t676+t893+t946;
t1001 = t104+t434+t560+t681+t903+t951;
t1003 = t118+t470+t575+t683+t908+t955;
t1004 = t669.*t1002;
t1013 = t941.*t963;
t1016 = -t1015;
t1018 = t668.*t1009;
t1021 = -t1020;
t1027 = t963.*t977;
t1029 = -t1028;
t1032 = -t1031;
t1038 = t985.*t1000;
t1044 = t130+t497+t598+t682+t686+t909+t911+t952+t958;
t1045 = t129+t496+t597+t683+t685+t908+t912+t955+t956;
t1058 = -t1057.*(t228-t306);
t1059 = t1057.*(t228-t306);
t1065 = t979+t1033+t1034;
t999 = t58+t336+t520+t675+t892+t948;
t1005 = t669.*t1003;
t1014 = -t1013;
t1039 = t985.*t1001;
t1040 = -t1038;
t1042 = t990.*t998;
t1046 = t998.*t1001;
t1049 = t771.*t1045;
t1050 = -t1044.*(t486-t674);
t1051 = t959+t981+t1018;
t1055 = t717+t793+t1012+t1016;
t1056 = t640+t715+t1027+t1029;
t1061 = t995+t997+t1004;
t1066 = t299.*t1065;
t1006 = -t1005;
t1041 = -t1039;
t1043 = t990.*t999;
t1047 = t999.*t1000;
t1048 = -t1046;
t1052 = t622.*t1051;
t1054 = t718+t795+t1011+t1014;
t1062 = t699.*t1061;
t1063 = (t303+t17.*(t228-t306)).*(-t996+t1005+t991.*(t486-t674));
t1067 = -t1066;
t1068 = t788+t864+t1040+t1042;
t1070 = t1049+t1050;
t1053 = -t1052;
t1060 = t994+t996+t1006;
t1064 = -t1062;
t1069 = t790+t863+t1041+t1043;
t1071 = t622.*t1070;
t1073 = t716+t794+t1047+t1048;
t1072 = -t1071;
et1 = t23.*(-4.710919801360536e-3)-t28.*2.43593206408921e-2+t938+t939+t989+t1021+t1024+t1032+t1053+t1059+t1063+t1064+t1067+t1072-t964.*(t133+t484+t638+t729);
et2 = (t1038-t1042+t27.*(t30.*(t248-t249)+t25.*(t358-t617)).*7.26735e-3+t32.*(t31.*(t705+t25.*(t248-t249))+t26.*(t349-t618)).*7.26735e-3).*(t254+t391+t626+t17.*t873-t21.*t940)+t1069.*(t250+t390+t627+t21.*t873+t17.*t940);
et3 = (t23.*t24.*1.999853847e-1-t28.*t29.*1.999853847e-1).*(t43-t59+2.243335e-2);
et4 = dq1.*t2.*(-2.63818724e-8)+(-t1027+t1028+t30.*(t248-t249).*1.08769e-2+t25.*(t358-t617).*1.08769e-2).*(t259+t267+t392+t394+t873)-t1073.*(t98+t234+t386+t387+t388+t645+t646+t825+t871);
et5 = -t1054.*(t140+t258+t270+t388+t398+t825+t871)-(t23.*t29.*1.999853847e-1+t24.*t28.*1.999853847e-1).*(t112+1.580661e-2)-t1037.*(t141+t153+t266+t276+t822);
et6 = (-t967+t968+t30.*(t248-t249).*2.889644e-2+t25.*(t358-t617).*2.889644e-2).*(t137+t273+t710+t801-t19.*t55.*t78.*3.790634411375469e-18);
et7 = (t135+t800).*(t405-t628-t875+t876)-(-t1012+t1015+t31.*(t705+t25.*(t248-t249)).*1.08769e-2+t26.*(t349-t618).*1.08769e-2).*(t139+t255+t272+t395+t940);
et8 = t1036.*(t138+t252+t708+t802+t15.*t55.*t78.*3.790634411375469e-18)-(t310+t315+t55.*t78.*6.374153504905841e-18).*(t297-t300+t916-t917);
et9 = t938+t939+t989+t1021+t1024+t1032+t1053+t1059+t1063+t1064+t1067+t1072+(-t967+t968+t30.*(t248-t249).*2.889644e-2+t25.*(t358-t617).*2.889644e-2).*(t137+t273+t730-t19.*t55.*t78.*8.66274921222547e-18);
et10 = (t1038-t1042+t27.*(t30.*(t248-t249)+t25.*(t358-t617)).*7.26735e-3+t32.*(t31.*(t705+t25.*(t248-t249))+t26.*(t349-t618)).*7.26735e-3).*(t254+t391+t626+t17.*t782-t21.*t868)-t964.*(t133+t729)+t1069.*(t250+t390+t627+t21.*t782+t17.*t868);
et11 = (-t1027+t1028+t30.*(t248-t249).*1.08769e-2+t25.*(t358-t617).*1.08769e-2).*(t259+t267+t392+t394+t782)-t1073.*(t98+t234+t386+t387+t388+t645+t646+t776+t783)+t23.*t24.*4.486342129859745e-3;
et12 = t23.*t29.*(-3.161090981652867e-3)-t24.*t28.*3.161090981652867e-3;
et13 = t28.*t29.*(-4.486342129859745e-3)-t1054.*(t140+t258+t270+t388+t398+t776+t783)+t1036.*(t138+t252+t731+t15.*t55.*t78.*8.66274921222547e-18)-t1037.*(t141+t153+t266+t276+t773);
et14 = (t135+t728).*(t405-t628-t875+t876)-(-t1012+t1015+t31.*(t705+t25.*(t248-t249)).*1.08769e-2+t26.*(t349-t618).*1.08769e-2).*(t139+t255+t272+t395+t868);
et15 = t55.*t78.*(t297-t300+t916-t917).*(-6.374153504905841e-18);
et16 = t19.*3.251444605336828e-2+3.306395640309251e-6;
et17 = -t967+t968+t30.*(t248-t249).*2.889644e-2+t25.*(t358-t617).*2.889644e-2;
et18 = t15.*5.157359871151559e-3+t110+t15.*t17.*1.580624215070616e-2+t15.*t21.*8.5910527129662e-3;
et19 = t17.*t126.*(-9.99471e-3)+t21.*t126.*1.838876e-2;
et20 = t16.*(-6.373432765934105e-3)+t19.*4.990257941055339e-2;
et21 = t20.*2.906183788415621e-3+t16.*t19.*4.888197259476159e-3;
et22 = t19.*t20.*1.07201054193752e-2;
et23 = t15.*1.07201054193752e-2-t20.*3.311505989057797e-5;
et24 = t15.*t20.*4.990257941055339e-2-t16.*t19.*5.569948660843684e-5;
et25 = t20.*9.397297665331243e-3+t16.*t19.*1.580624215070616e-2;
et26 = t17.*t19.*4.990257941055339e-2+t17.*t122.*(3.0./5.0e+2)+t15.*t20.*t21.*4.990257941055339e-2;
et27 = t20.*5.107645374058002e-3+t16.*t19.*8.5910527129662e-3;
et28 = t19.*t21.*4.990257941055339e-2+t21.*t122.*(3.0./5.0e+2)-t15.*t17.*t20.*4.990257941055339e-2;
et29 = t15.*4.888197259476159e-3-t16.*3.311505989057797e-5+t110;
et30 = t19.*t20.*5.569948660843684e-5;
et31 = t796.*(-8.595599785252598e-1)+t797.*5.110348748545983e-1-t798.*8.595599785252598e-1+t799.*5.110348748545983e-1+t865.*5.110348748545983e-1;
et32 = t866.*8.595599785252598e-1+t916.*2.688673858077708e-3-t917.*2.688673858077708e-3;
et33 = t929.*(-5.110348748545983e-1)+t931.*5.110348748545983e-1+t924.*(t96+t292).*5.110348748545983e-1+et16.*et17+t1073.*(et18+et19);
et34 = (-t1027+t1028+t30.*(t248-t249).*1.08769e-2+t25.*(t358-t617).*1.08769e-2).*(et20+et21+et22)+t15.*t1019.*8.595599785252598e-1-t19.*t1030.*8.595599785252598e-1;
et35 = t15.*t1065.*8.595599785252598e-1-t122.*t1051+t126.*t1057-t122.*t1070+(et23+et24).*(-t1012+t1015+t31.*(t705+t25.*(t248-t249)).*1.08769e-2+t26.*(t349-t618).*1.08769e-2);
et36 = (t1038-t1042+t27.*(t30.*(t248-t249)+t25.*(t358-t617)).*7.26735e-3+t32.*(t31.*(t705+t25.*(t248-t249))+t26.*(t349-t618)).*7.26735e-3).*(et25+et26)-(t15.*t21.*8.595599785252598e-1-t17.*t126).*(-t996+t1005+t991.*(t486-t674))+t1069.*(et27+et28);
et37 = -t1037.*(t15.*5.561353061058431e-6+t19.*5.023973353684009e-3)+t1054.*(et29+et30)+t1061.*(t15.*t17.*8.595599785252598e-1+t21.*t126);
et38 = -t1036.*(t15.*3.251444605336828e-2-2.986906857247653e-3);
et39 = t40.*t55.*t80.*5.091703513734173e-22;
et40 = t41.*t55.*t80.*(-8.564238525144865e-22);
et41 = t706.*1.688944904408e-4-t929+t931-t967.*6.47e-6+t968.*6.47e-6+t970.*5.84482e-3;
et42 = t971.*(-5.84482e-3);
et43 = (t20.*1.838876e-2+t17.*t20.*(3.0./5.0e+2)).*(t1038-t1042+t27.*(t30.*(t248-t249)+t25.*(t358-t617)).*7.26735e-3+t32.*(t31.*(t705+t25.*(t248-t249))+t26.*(t349-t618)).*7.26735e-3)+t924.*(t96+t292);
et44 = -t1073.*(t16.*t17.*9.99471e-3-t16.*t21.*1.838876e-2)-t16.*t1054.*6.48e-5-t20.*t1051+t16.*t1057-t20.*t1070;
et45 = -(t16.*1.247162e-2-t20.*5.68686e-3).*(-t1027+t1028+t30.*(t248-t249).*1.08769e-2+t25.*(t358-t617).*1.08769e-2);
et46 = t25.*(t248-t249).*(-1.688944904408e-4)+t30.*(t248-t249).*1.869599668e-7;
et47 = t25.*(t358-t617).*1.869599668e-7;
et48 = t20.*(-t1012+t1015+t31.*(t705+t25.*(t248-t249)).*1.08769e-2+t26.*(t349-t618).*1.08769e-2).*(-6.48e-5)+t1069.*(t20.*9.99471e-3+t20.*t21.*(3.0./5.0e+2));
et49 = t16.*t17.*(-t996+t1005+t991.*(t486-t674))+t16.*t21.*t1061;
et50 = t1011.*(-5.68686e-3)+t1012.*1.247162e-2+t1013.*5.68686e-3-t1015.*1.247162e-2-t1065;
et51 = t26.*(t705+t25.*(t248-t249)).*(-6.1855407534e-5)-t31.*(t705+t25.*(t248-t249)).*1.35652563578e-4;
et52 = -t1073.*(t17.*1.838876e-2+t21.*9.99471e-3+3.0./5.0e+2)-t17.*t1061-t26.*(t349-t618).*1.35652563578e-4;
et53 = t31.*(t349-t618).*6.1855407534e-5+t21.*(-t996+t1005+t991.*(t486-t674));
et54 = t1038.*1.838876e-2-t1039.*9.99471e-3-t1042.*1.838876e-2+t1043.*9.99471e-3-t1049;
et55 = t27.*(t30.*(t248-t249)+t25.*(t358-t617)).*1.33637554986e-4+t32.*(t30.*(t248-t249)+t25.*(t358-t617)).*7.26350557185e-5+t1044.*(t486-t674);
et56 = t27.*(t31.*(t705+t25.*(t248-t249))+t26.*(t349-t618)).*(-7.26350557185e-5)+t32.*(t31.*(t705+t25.*(t248-t249))+t26.*(t349-t618)).*1.33637554986e-4;
h = [et1+et2+et3+et4+et5+et6+et7+et8;et9+et10+et11+et12+et13+et14+et15;et31+et32+et33+et34+et35+et36+et37+et38+et39+et40;et41+et42+et43+et44+et45+et46+et47+et48+et49;et50+et51+et52+et53;et54+et55+et56];
h = real(h);
end
